simulink model "modelo_f_CAPTURAS_FINALES"  (R2024b)
settings: Solver=ode15s  StartTime=0.0  StopTime=50  FixedStep=T_s  RelTol=1e-3
InitFcn:
  | clc
  | clear
  | close all
  | clear all
  | clear mex
  | parametros
  | gain_CL
  | calculo_observador_carro
  | calculo_observador_izaje
values from neighbouring files (symbols this model uses):
  b_cx = 1e6    (= 1000000)    [parametros.m]
  b_cy = 1e7    (= 10000000)    [parametros.m]
  b_hb = 1e8    (= 100000000)    [parametros.m]
  b_hd = 8    [parametros.m]
  b_hm = 18    [parametros.m]
  b_t = 90    [parametros.m]
  b_ta = M_tEq*w_des_t*(1+n_t+n_t^2)-b_tEq    [gain_CL.m]
  b_tb = 5e6    (= 5000000)    [parametros.m]
  b_td = 1.8    [parametros.m]
  b_tm = 6    [parametros.m]
  b_tw = 3e3    (= 3000)    [parametros.m]
  b_wu = 150    [parametros.m]
  container_pillars = container_pillars(randperm(19))    [parametros.m]
  dx_grid_lidar = 0.01    [parametros.m]
  escenario = 1    [parametros.m]
  g = 9.80665    [parametros.m]
  H_c = 2.59    [parametros.m]
  H_truck = 1    [parametros.m]
  i_h = 22    [parametros.m]
  i_t = 30    [parametros.m]
  J_hd_hEb = 3800    [parametros.m]
  J_hm_hb = 30    [parametros.m]
  J_td = 1200    [parametros.m]
  J_tm_tb = 7    [parametros.m]
  K_cy = 1.8e9    (= 1800000000)    [parametros.m]
  k_tsa = M_tEq*w_des_t^2*n_t*(1+n_t+n_t^2)    [gain_CL.m]
  k_tsia = M_tEq*w_des_t^3*n_t^3    [gain_CL.m]
  K_tw = 4.8e5    (= 480000)    [parametros.m]
  k_wu = 2.36e8    (= 236000000)    [parametros.m]
  Kp_ext_carro = 0.11    [gain_CL.m]
  Kp_ext_izaje = 0.5    [gain_CL.m]
  l_h0 = (Y_t0-y_l0)    (= 15)    [parametros.m]
  l_h_max = Y_t0-y_h_min    (= 65)    [parametros.m]
  l_h_maxE = l_h_max+0.5    (= 65.5)    [parametros.m]
  l_h_min = Y_t0-y_h_max    (= 5)    [parametros.m]
  l_h_minE = l_h_min-0.5    (= 4.5)    [parametros.m]
  Lt = place(At', Ct', polos_deseados)'    [calculo_observador_carro.m]
  M_cmax = 50000    [parametros.m]
  M_cmin = 2000    [parametros.m]
  M_s = 15000    [parametros.m]
  M_t = 30000    [parametros.m]
  r_hd = 0.75    [parametros.m]
  r_td = 0.50    (= 0.5)    [parametros.m]
  T_hbMax = 5e4    (= 50000)    [parametros.m]
  T_hEbMax = 1.1e6    (= 1100000)    [parametros.m]
  T_hmMax = 2e4    (= 20000)    [parametros.m]
  T_s = 0.001    [parametros.m]
  T_s0 = 0.001    [parametros.m]
  T_s1 = 0.020    (= 0.02)    [parametros.m]
  T_s2 = 0.020    (= 0.02)    [parametros.m]
  T_tbMax = 5e3    (= 5000)    [parametros.m]
  T_tmMax = 4e3    (= 4000)    [parametros.m]
  tau_tm = 1e-3    (= 0.001)    [parametros.m]
  theta_hm0 = -l_h0*i_h*2/r_hd    (= -880)    [parametros.m]
  theta_tm0 = (x_t0)*i_t/r_td    (= -1500)    [parametros.m]
  trucks0 = [0, 0, 0, 0, 0]    [parametros.m]
  v_h_max_load = 1.5    [parametros.m]
  v_h_max_noload = 3    [parametros.m]
  v_lx0 = 0    [parametros.m]
  v_ly0 = 0    [parametros.m]
  v_t0 = 0    [parametros.m]
  v_t_max = 4    [parametros.m]
  W_c = ctrb(A, B_c(:,1))    [CyO_carro.m]    (also in CyO_izaje.m; parametros.m = 2.44)
  w_hm0 = 0    [parametros.m]
  w_hm_min_BRK = 0.005    [parametros.m]
  w_hm_rated = v_h_max_load*2*i_h/r_hd    (= 88)    [parametros.m]
  w_tm0 = (v_t0)*i_t/r_td    (= 0)    [parametros.m]
  w_tm_min_BRK = 0.005    [parametros.m]
  x_c0_left = -35    [parametros.m]
  x_c0_right = 55    [parametros.m]
  x_containers_left_lim = 1.5    [parametros.m]
  x_containers_right_lim = 48.5    [parametros.m]
  x_l0 = x_t0    (= -25)    [parametros.m]
  x_lidar_offset = 3.0    (= 3)    [parametros.m]
  x_t0 = -25    [parametros.m]
  x_t_max = 50    [parametros.m]
  x_t_maxE = x_t_max+0.5    (= 50.5)    [parametros.m]
  x_t_min = -30    [parametros.m]
  x_t_minE = x_t_min-0.5    (= -30.5)    [parametros.m]
  y_h_min = -20    [parametros.m]
  y_l0 = 30    [parametros.m]
  Y_sb = 5.0    (= 5)    [parametros.m]
  Y_t0 = 45    [parametros.m]
undefined symbols (not defined in the file or in its folder): Lh, parametros
libraries: dspnetwork x2, dspsigops x1, simulink x1
(part 2 of 5)

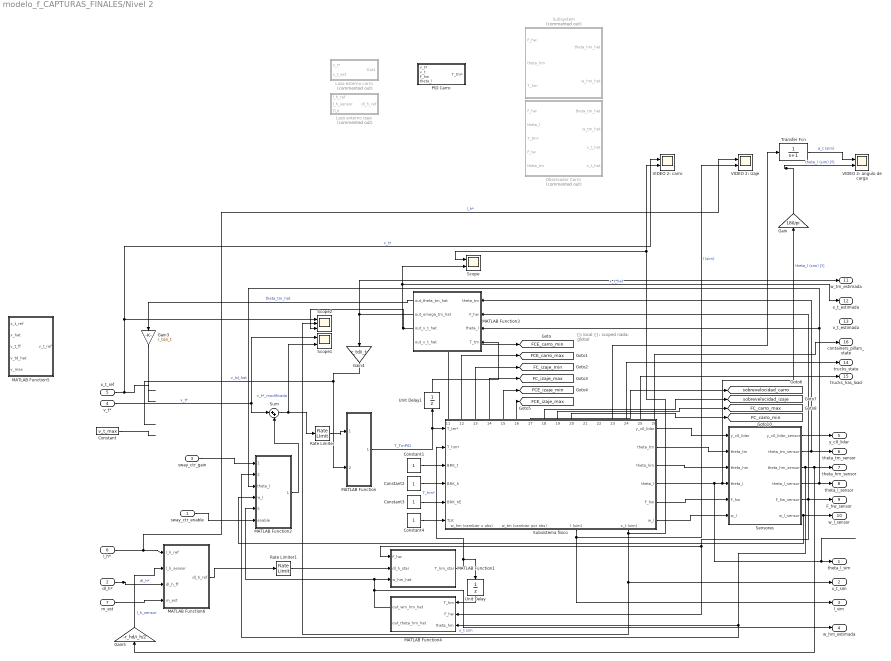
== system modelo_f_CAPTURAS_FINALES/Nivel 2 ==
  note: []: local
      | {}: scoped
      | nada: global
  sway_ctr_enable : Inport
  dl_h* : Inport  Port=2
  sway_ctr_gain : Inport  Port=3
  v_t* : Inport  Port=4
  x_t_ref : Inport  Port=5
  l_h* : Inport  Port=6
  m_est : Inport  Port=7
  Constant : Constant  Value=v_t_max
  Constant{1..4} (4 alike) : Constant
  Gain : Gain  Gain=180/pi
  Gain3 : Gain  Gain=r_td/i_t
  Gain4 : Gain  Gain=r_td/i_t
  Gain5 : Gain  Gain=-r_hd/i_h/2
  Lazo externo carro : Subsystem  Commented=on
  Lazo externo izaje : Subsystem  Commented=on
  MATLAB Function : MATLAB Function  TreatAsAtomicUnit=on  SystemSampleTime=T_s0
  MATLAB Function1 : MATLAB Function  TreatAsAtomicUnit=on  SystemSampleTime=T_s0
  MATLAB Function2 : MATLAB Function  TreatAsAtomicUnit=on  SystemSampleTime=T_s0
  MATLAB Function3 : MATLAB Function  TreatAsAtomicUnit=on  SystemSampleTime=T_s0
  MATLAB Function4 : MATLAB Function  TreatAsAtomicUnit=on  SystemSampleTime=T_s0
  MATLAB Function5 : MATLAB Function  TreatAsAtomicUnit=on
  MATLAB Function6 : MATLAB Function  TreatAsAtomicUnit=on
  Observador Carro : Subsystem  Commented=on
  PID Carro : Subsystem
  Rate Limiter : RateLimiter  RisingSlewLimit=0.8  FallingSlewLimit=-0.8  SampleTimeMode=inherited  InitialCondition=T_s
  Rate Limiter1 : RateLimiter  RisingSlewLimit=0.75  FallingSlewLimit=-0.75  SampleTimeMode=inherited  InitialCondition=T_s
  Scope : Scope  NumInputPorts=2
  Scope1 : Scope  NumInputPorts=2
  Scope2 : Scope  NumInputPorts=3
  Sensores : Subsystem
  Subsistema físico : Subsystem
      settings: PortSchema="{\"entries\":[{\"content\":{\"sides\":[{\"content\":{\"connectorIds\":[\"In1\",\"In2\",\"In3\",\"In4\",\"In5\",\"In6\"]},\"type\":\"ConnectorPlacement.EquallySpacedRectSide\",\"uuid\":\"aa1cb789-2051-45a4-8cb8-6dd2078290cc\"},{\"content\":{\"connectorIds\":[\"Out1\",\"Out2\",\"Out3\",\"Out4\",\"Out5\",\"Out6\"],\"side\":\"RIGHT\"},\"type\":\"ConnectorPlacement.EquallySpacedRectSide\",\"uuid\":\"7fe62279-dd3b-46db-ba9e-e4633dcea5c6\"},{\"content\":{\"connectorIds\":[\"Out11\",\"Out12\",\"Out13\",\"Out14\",\"Out15\",\"Out16\",\"Out17\",\"Out18\",\"Out19\",\"Out20\",\"Out21\",\"Out22\",\"Out23\",\"Out24\",\"Out25\",\"Out26\"],\"side\":\"TOP\"},\"type\":\"ConnectorPlacement.EquallySpacedRectSide\",\"uuid\":\"a5663ea7-10d8-47d7-b8ed-8fbfb239b85a\"},{\"content\":{\"connectorIds\":[\"Out7\",\"Out8\",\"Out9\",\"Out10\"],\"side\":\"BOTTOM\"},\"type\":\"ConnectorPlacement.EquallySpacedRectSide\",\"uuid\":\"9ec9131f-7b2f-42d7-8a86-9462c3c282b3\"}]},\"type\":\"ConnectorPlacement.EquallySpacedConnector\",\"uuid\":\"e7df1a56-7803-4e0d-8bf9-081877eb8c08\"}],\"packageUris\":[\"http://schema.mathworks.com/mf0/Connector/R2020b\"],\"version\":\"1.0\"}"
  Subsystem : Subsystem  Commented=on
  Sum : Sum  Inputs=|++
  Transfer Fcn : TransferFcn  Denominator=[1 1]
  Unit Delay : UnitDelay  SampleTime=T_s  HasFrameUpgradeWarning=on
  Unit Delay1 : UnitDelay  SampleTime=T_s  HasFrameUpgradeWarning=on
  VIDEO 2: angulo de carga : Scope  NumInputPorts=2
  VIDEO 2: carro : Scope  NumInputPorts=2
  VIDEO 2: izaje : Scope  NumInputPorts=2
  theta_l_sim : Outport
  x_t_sim : Outport  Port=2
  l_sim : Outport  Port=3
  w_hm_estimada : Outport  Port=4
  y_c0_lidar : Outport  Port=5
  theta_tm_sensor : Outport  Port=6
  theta_hm_sensor : Outport  Port=7
  theta_l_sensor : Outport  Port=8
  F_hw_sensor : Outport  Port=9
  w_l_sensor : Outport  Port=10
  w_tm_estimada : Outport  Port=11
  x_t_estimada : Outport  Port=12
  v_t_estimada : Outport  Port=13
  trucks_state : Outport  Port=14
  trucks_has_load : Outport  Port=15
  containers_pillars_state : Outport  Port=16
  tag scope: FCE_carro_max=global, FCE_carro_min=global, FCE_izaje_max=global, FCE_izaje_min=global, FC_carro_max=global, FC_carro_min=global, FC_izaje_max=global, FC_izaje_min=global, sobrevelocidad_carro=global, sobrevelocidad_izaje=global
  wires:
  Sensores/5(F_hw_sensor) -> F_hw_sensor/1, MATLAB Function4/2(F_hw), MATLAB Function1/1(F_hw), MATLAB Function3/2(F_hw)
  Sensores/2(theta_tm_sensor) -> theta_tm_sensor/1, MATLAB Function3/1(theta_tm)
  Subsistema físico/19(FC_carro_max) -> [FC_carro_max]
  Sensores/3(theta_hm_sensor) -> theta_hm_sensor/1, Gain5/1, MATLAB Function4/3(theta_hm), MATLAB Function2/2(theta_hm)
  Sensores/6(w_l_sensor) -> w_l_sensor/1, MATLAB Function2/4(w_l)
  Subsistema físico/15(FCE_izaje_min) -> [FCE_izaje_min]
  Unit Delay/1 -> MATLAB Function4/1(T_hm)
  Subsistema físico/13(FC_izaje_min) -> [FC_izaje_min]
  Subsistema físico/16(FCE_izaje_max) -> [FCE_izaje_max]
  MATLAB Function1/1(T_hm_star) -> Unit Delay/1, Subsistema físico/2(T_hm*)  "T_hm*"
  Subsistema físico/6(w_l) -> Sensores/6(w_l)
  Subsistema físico/17(sobrevelocidad_carro) -> [sobrevelocidad_carro]
  Subsistema físico/3(theta_hm) -> Sensores/3(theta_hm)
  MATLAB Function4/1(out_wm_hm_hat) -> MATLAB Function2/5(w_hm_hat), MATLAB Function1/3(w_hm_hat), w_hm_estimada/1
  dl_h*/1 -> MATLAB Function6/3(dl_h_ff)  "dl_h*"
  Subsistema físico/1(y_c0_lidar) -> Sensores/1(y_c0_lidar)
  Subsistema físico/5(F_hw) -> Sensores/5(F_hw)
  Subsistema físico/2(theta_tm) -> Sensores/2(theta_tm)
  Subsistema físico/18(sobrevelocidad_izaje) -> [sobrevelocidad_izaje]
  Subsistema físico/11(FCE_carro_min) -> [FCE_carro_min]
  Subsistema físico/4(theta_l) -> Gain/1, Sensores/4(theta_l), theta_l_sim/1  "theta_l (sim) [º]"
  Subsistema físico/14(FC_izaje_max) -> [FC_izaje_max]
  Subsistema físico/20(FC_carro_min) -> [FC_carro_min]
  Subsistema físico/12(FCE_carro_max) -> [FCE_carro_max]
  Constant1/1 -> Subsistema físico/3(BRK_t)
  Constant2/1 -> Subsistema físico/4(BRK_h)
  Constant3/1 -> Subsistema físico/5(BRK_hE)
  Constant4/1 -> Subsistema físico/6(TLK)
  Sensores/1(y_c0_lidar_sensor) -> y_c0_lidar/1
  sway_ctr_enable/1 -> MATLAB Function2/6(enable)
  MATLAB Function3/2(out_omega_tm_hat) -> w_tm_estimada/1, Gain4/1
  Gain4/1 -> MATLAB Function/2(v_td_hat)  "v_td_hat"
  v_t*/1 -> Sum/1, Scope1/1  "v_t*"
  Sensores/4(theta_l_sensor) -> theta_l_sensor/1, MATLAB Function2/3(theta_l), MATLAB Function3/3(theta_l)
  Unit Delay1/1 -> MATLAB Function3/4(T_tm)
  Subsistema físico/10(x_t (sim)) -> Scope2/2, x_t_sim/1, Scope/1, VIDEO 2: carro/2  "x_t sim"
  Subsistema físico/9(l (sim)) -> VIDEO 2: izaje/2, l_sim/1  "l (sim)"
  MATLAB Function3/3(out_x_t_hat) -> Scope2/3, Scope/2, x_t_estimada/1  "x_t_hat"
  MATLAB Function3/1(out_theta_tm_hat) -> Gain3/1  "theta_tm_hat"
  Subsistema físico/24(trucks_state) -> trucks_state/1
  x_t_ref/1 -> Scope2/1, VIDEO 2: carro/1  "x_t*"
  sway_ctr_gain/1 -> MATLAB Function2/1(sway_ctr_gain)
  Subsistema físico/25(trucks_has_load) -> trucks_has_load/1
  MATLAB Function/1(T_tm_star) -> Unit Delay1/1, Subsistema físico/1(T_tm*)  "T_TmPID"
  MATLAB Function2/1(v_balanceo) -> Sum/2
  Sum/1 -> Scope1/2, Rate Limiter/1  "v_t*_modificada"
  Constant/1 -> ?
  Gain3/1 -> ?
  Gain5/1 -> MATLAB Function6/2(l_h_sensor)  "l_h_sensor"
  l_h*/1 -> VIDEO 2: izaje/1, MATLAB Function6/1(l_h_ref)  "l_h*"
  MATLAB Function6/1(dl_h_ref) -> Rate Limiter1/1
  Rate Limiter/1 -> MATLAB Function/1(v_t_star)
  Rate Limiter1/1 -> MATLAB Function1/2(dl_h_star)
  Subsistema físico/26(containers_pillars_state) -> containers_pillars_state/1
  m_est/1 -> MATLAB Function6/4(m_est)
  Gain/1 -> VIDEO 2: angulo de carga/2  "theta_l (sim) [º]"
  Subsistema físico/23(a_t(sim)) -> Transfer Fcn/1
  Transfer Fcn/1 -> VIDEO 2: angulo de carga/1  "a_t (sim)"

== system modelo_f_CAPTURAS_FINALES/UDP: Controller reader ==
  Cast To Boolean{,2..5} (5 alike) : DataTypeConversion  OutDataTypeStr=boolean  SaturateOnIntegerOverflow=off  RndMeth=Floor
  MATLAB Function : MATLAB Function  TreatAsAtomicUnit=on
  UDP Receive1 : dspnetwork/UDP Receive  localURL='0.0.0.0'  localPort=5005  remoteURL='0.0.0.0'  remotePort=-1  recvBufferSize=14  dims=255  signalDatatype=uint8  isComplex=off  isVarSize=on  showBlockingTime=off  blockingTime=0  sampletime=1  blockPlatform=[]
      settings: LibrarySourceBlock=dspsrcs4/UDP Receive
  tag scope: JS_emgy_ack_cmd=global, JS_emgy_cmd=global, JS_hoist_cmd=global, JS_sway_ctrl_cmd=global, JS_system_enable=global, JS_tlk_cmd=global, JS_trolley_cmd=global
  wires:
  UDP Receive1/1 -> MATLAB Function/1(data)
  MATLAB Function/1(trolley_cmd) -> [JS_trolley_cmd]  "trolley_cmd"
  MATLAB Function/2(hoist_cmd) -> [JS_hoist_cmd]  "hoist_cmd"
  MATLAB Function/3(system_on) -> Cast To Boolean/1  "system_on"
  MATLAB Function/4(twistlock) -> Cast To Boolean2/1  "twistlock"
  MATLAB Function/5(sway_ctrl) -> Cast To Boolean3/1  "sway_ctrl"
  MATLAB Function/6(emergency) -> Cast To Boolean4/1  "emergency"
  MATLAB Function/7(emgy_ack) -> Cast To Boolean5/1  "emgy ack"
  Cast To Boolean/1 -> [JS_system_enable]
  Cast To Boolean2/1 -> [JS_tlk_cmd]
  Cast To Boolean4/1 -> [JS_emgy_cmd]
  Cast To Boolean5/1 -> [JS_emgy_ack_cmd]
  Cast To Boolean3/1 -> [JS_sway_ctrl_cmd]

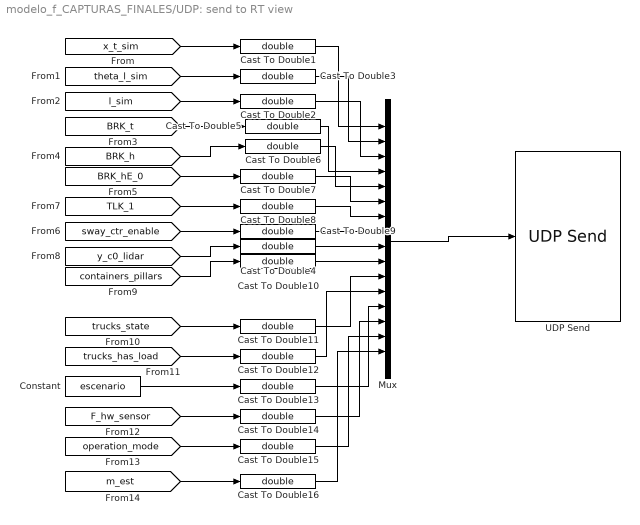
== system modelo_f_CAPTURAS_FINALES/UDP: send to RT view ==
  Cast To Double{1..16} (16 alike) : DataTypeConversion  OutDataTypeStr=double  SaturateOnIntegerOverflow=off  RndMeth=Floor
  Constant : Constant  Value=escenario
  Mux : Mux  Inputs=16
  UDP Send : dspnetwork/UDP Send  remoteURL='127.0.0.1'  remotePort=5010  localURL='0.0.0.0'  localPortSource=Automatically determine  localPort=-1  sendBufferSize=8192  sampletime=-1  blockPlatform=[]  separateLengthPort=0
      settings: LibrarySourceBlock=dspsnks4/UDP Send
  wires:
  [x_t_sim] -> Cast To Double1/1
  [theta_l_sim] -> Cast To Double3/1
  Mux/1 -> UDP Send/1
  [l_sim] -> Cast To Double2/1
  [BRK_t] -> Cast To Double5/1
  [BRK_h] -> Cast To Double6/1
  [BRK_hE_0] -> Cast To Double7/1
  [sway_ctr_enable] -> Cast To Double9/1
  [TLK_1] -> Cast To Double8/1
  Cast To Double1/1 -> Mux/1
  Cast To Double3/1 -> Mux/2
  Cast To Double2/1 -> Mux/3
  Cast To Double5/1 -> Mux/4
  Cast To Double6/1 -> Mux/5
  Cast To Double7/1 -> Mux/6
  Cast To Double8/1 -> Mux/7
  Cast To Double9/1 -> Mux/8
  [y_c0_lidar] -> Cast To Double4/1
  Cast To Double4/1 -> Mux/9
  [containers_pillars] -> Cast To Double10/1
  Cast To Double10/1 -> Mux/10
  [trucks_state] -> Cast To Double11/1
  Cast To Double11/1 -> Mux/11
  [trucks_has_load] -> Cast To Double12/1
  Cast To Double12/1 -> Mux/12
  Cast To Double13/1 -> Mux/13
  Constant/1 -> Cast To Double13/1
  Cast To Double14/1 -> Mux/14
  [F_hw_sensor] -> Cast To Double14/1
  [operation_mode] -> Cast To Double15/1
  Cast To Double15/1 -> Mux/15
  [m_est] -> Cast To Double16/1
  Cast To Double16/1 -> Mux/16

== system modelo_f_CAPTURAS_FINALES/Nivel 2/Lazo externo carro ==
  "x_t* " : Inport
  x_t_est : Inport  Port=2
  Gain : Gain  Gain=Kp_ext_carro
  Saturation : Saturate  UpperLimit=v_t_max  LowerLimit=-v_t_max
  Sum : Sum  Inputs=|+-
  Out1 : Outport
  wires:
  "x_t* "/1 -> Sum/1
  x_t_est/1 -> Sum/2
  Sum/1 -> Gain/1
  Gain/1 -> Saturation/1
  Saturation/1 -> Out1/1

== system modelo_f_CAPTURAS_FINALES/Nivel 2/Lazo externo izaje ==
  "l_h_ref " : Inport
  l_h_sensor : Inport  Port=2
  TLK : Inport  Port=3
  Gain : Gain  Gain=Kp_ext_izaje
  Sum : Sum  Inputs=|+-
  Switch : Switch  Criteria=u2 ~= 0  SaturateOnIntegerOverflow=off  InputSameDT=off
  loaded : Saturate  UpperLimit=v_h_max_load  LowerLimit=-v_h_max_load
  no load : Saturate  UpperLimit=v_h_max_noload  LowerLimit=-v_h_max_noload
  dl_h_ref : Outport
  wires:
  "l_h_ref "/1 -> Sum/1
  l_h_sensor/1 -> Sum/2
  Sum/1 -> Gain/1
  Gain/1 -> no load/1, loaded/1
  TLK/1 -> Switch/2
  loaded/1 -> Switch/1
  no load/1 -> Switch/3
  Switch/1 -> dl_h_ref/1

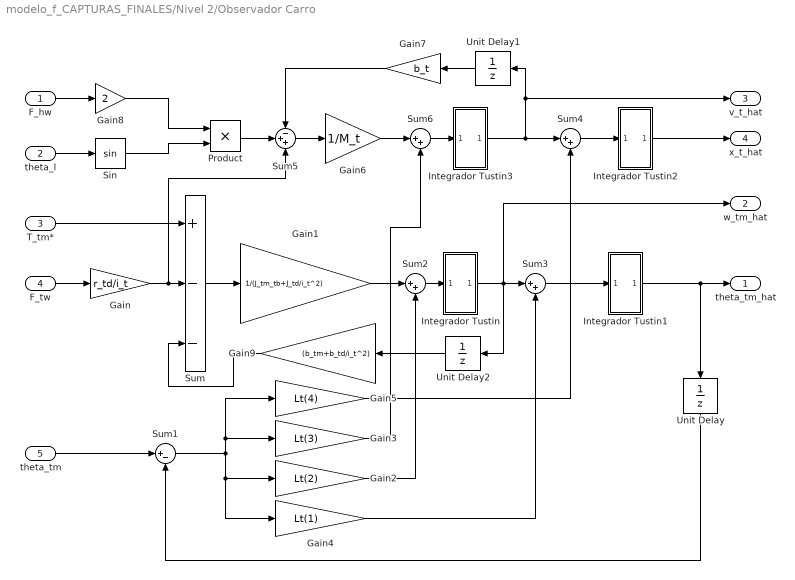
== system modelo_f_CAPTURAS_FINALES/Nivel 2/Observador Carro ==
  F_hw : Inport
  theta_l : Inport  Port=2
  T_tm* : Inport  Port=3
  F_tw : Inport  Port=4
  theta_tm : Inport  Port=5
  Gain : Gain  Gain=r_td/i_t
  Gain1 : Gain  Gain=1/(J_tm_tb+J_td/i_t^2)
  Gain2 : Gain  Gain=Lt(2)
  Gain3 : Gain  Gain=Lt(3)
  Gain4 : Gain  Gain=Lt(1)
  Gain5 : Gain  Gain=Lt(4)
  Gain6 : Gain  Gain=1/M_t
  Gain7 : Gain  Gain=b_t
  Gain8 : Gain  Gain=2
  Gain9 : Gain  Gain=(b_tm+b_td/i_t^2)
  Integrador Tustin : Subsystem
  Integrador Tustin1 : Subsystem
  Integrador Tustin2 : Subsystem
  Integrador Tustin3 : Subsystem
  Product : Product
  Sin : Trigonometry
  Sum : Sum  Inputs=+--
  Sum1 : Sum  Inputs=|+-
  Sum{2..4,6} (4 alike) : Sum  Inputs=|++
  Sum5 : Sum  Inputs=-++
  Unit Delay : UnitDelay  SampleTime=T_s1  HasFrameUpgradeWarning=on
  Unit Delay1 : UnitDelay  SampleTime=T_s1  HasFrameUpgradeWarning=on
  Unit Delay2 : UnitDelay  SampleTime=T_s1  HasFrameUpgradeWarning=on
  theta_tm_hat : Outport
  w_tm_hat : Outport  Port=2
  v_t_hat : Outport  Port=3
  x_t_hat : Outport  Port=4
  wires:
  T_tm*/1 -> Sum/1
  F_tw/1 -> Gain/1
  Gain/1 -> Sum5/3, Sum/2
  theta_tm/1 -> Sum1/1
  Integrador Tustin1/1(out) -> theta_tm_hat/1, Unit Delay/1
  Sum/1 -> Gain1/1
  Gain1/1 -> Sum2/1
  Sum2/1 -> Integrador Tustin/1(in)
  Sum3/1 -> Integrador Tustin1/1(in)
  Sum1/1 -> Gain5/1, Gain3/1, Gain2/1, Gain4/1
  Gain4/1 -> Sum3/2
  Gain2/1 -> Sum2/2
  Integrador Tustin/1(out) -> Unit Delay2/1, w_tm_hat/1, Sum3/1
  Integrador Tustin2/1(out) -> x_t_hat/1
  Sum4/1 -> Integrador Tustin2/1(in)
  Integrador Tustin3/1(out) -> Unit Delay1/1, v_t_hat/1, Sum4/1
  Gain5/1 -> Sum4/2
  Sum5/1 -> Gain6/1
  Gain7/1 -> Sum5/1
  Product/1 -> Sum5/2
  theta_l/1 -> Sin/1
  F_hw/1 -> Gain8/1
  Gain8/1 -> Product/1
  Sin/1 -> Product/2
  Gain9/1 -> Sum/3
  Unit Delay/1 -> Sum1/2
  Gain6/1 -> Sum6/1
  Sum6/1 -> Integrador Tustin3/1(in)
  Gain3/1 -> Sum6/2
  Unit Delay1/1 -> Gain7/1
  Unit Delay2/1 -> Gain9/1

== system modelo_f_CAPTURAS_FINALES/Nivel 2/PID Carro ==
  v_t* : Inport
  v_t : Inport  Port=2
  F_hw : Inport  Port=3
  theta_l : Inport  Port=4
  Gain : Gain  Gain=k_tsa
  Gain1 : Gain  Gain=k_tsia
  Gain2 : Gain  Gain=b_ta
  Gain3 : Gain  Gain=2
  Integrador Tustin1 : Subsystem
  Integrador Tustin2 : Subsystem
  Product : Product
  Sin : Trigonometry
  Sum : Sum  Inputs=|+-
  Sum1 : Sum  Inputs=+++
  Sum2 : Sum  Inputs=|+-
  T_tm* : Outport
  wires:
  v_t*/1 -> Sum/1
  v_t/1 -> Sum/2
  Sum/1 -> Gain2/1, Integrador Tustin1/1(in)
  Integrador Tustin1/1(out) -> Gain/1, Integrador Tustin2/1(in)
  Gain/1 -> Sum1/2
  Integrador Tustin2/1(out) -> Gain1/1
  Gain1/1 -> Sum1/1
  Gain2/1 -> Sum1/3
  Sum1/1 -> Sum2/1
  F_hw/1 -> Gain3/1
  theta_l/1 -> Sin/1
  Gain3/1 -> Product/1
  Sin/1 -> Product/2
  Product/1 -> Sum2/2
  Sum2/1 -> T_tm*/1

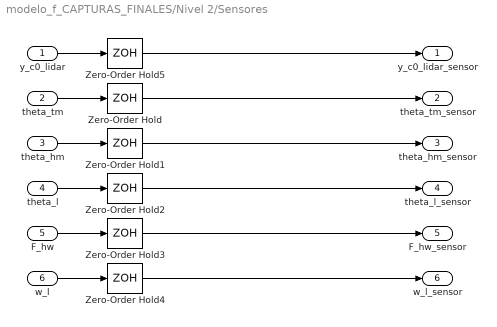
== system modelo_f_CAPTURAS_FINALES/Nivel 2/Sensores ==
  y_c0_lidar : Inport
  theta_tm : Inport  Port=2
  theta_hm : Inport  Port=3
  theta_l : Inport  Port=4
  F_hw : Inport  Port=5
  w_l : Inport  Port=6
  Zero-Order Hold{,2..5} (5 alike) : ZeroOrderHold  SampleTime=T_s
  Zero-Order Hold1 : ZeroOrderHold  SampleTime=T_s2
  y_c0_lidar_sensor : Outport
  theta_tm_sensor : Outport  Port=2
  theta_hm_sensor : Outport  Port=3
  theta_l_sensor : Outport  Port=4
  F_hw_sensor : Outport  Port=5
  w_l_sensor : Outport  Port=6
  wires:
  theta_tm/1 -> Zero-Order Hold/1
  Zero-Order Hold/1 -> theta_tm_sensor/1
  Zero-Order Hold1/1 -> theta_hm_sensor/1
  theta_hm/1 -> Zero-Order Hold1/1
  w_l/1 -> Zero-Order Hold4/1
  F_hw/1 -> Zero-Order Hold3/1
  theta_l/1 -> Zero-Order Hold2/1
  Zero-Order Hold2/1 -> theta_l_sensor/1
  Zero-Order Hold3/1 -> F_hw_sensor/1
  Zero-Order Hold4/1 -> w_l_sensor/1
  Zero-Order Hold5/1 -> y_c0_lidar_sensor/1
  y_c0_lidar/1 -> Zero-Order Hold5/1

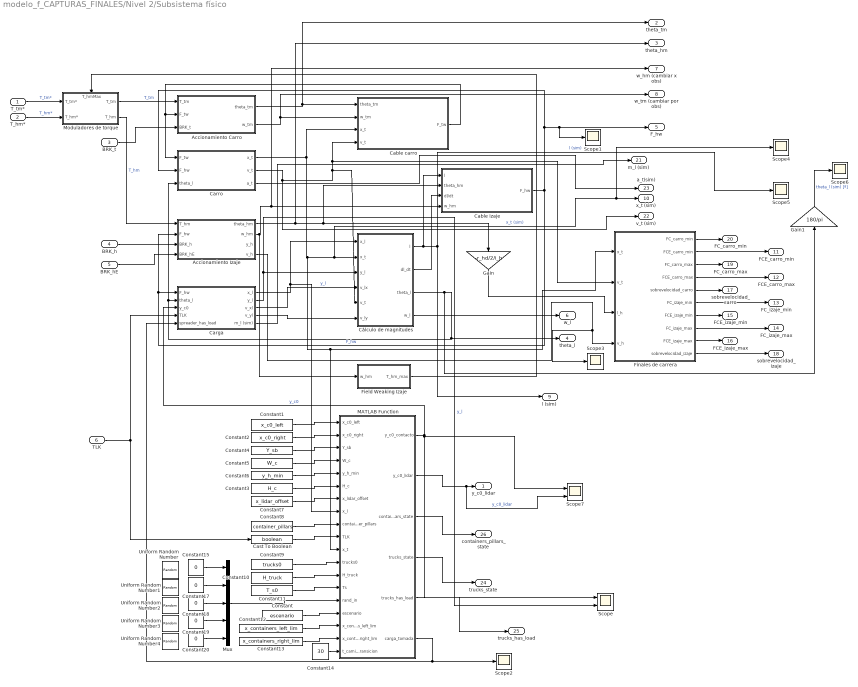
== system modelo_f_CAPTURAS_FINALES/Nivel 2/Subsistema físico ==
  T_tm* : Inport
  T_hm* : Inport  Port=2
  BRK_t : Inport  Port=3
  BRK_h : Inport  Port=4
  BRK_hE : Inport  Port=5
  TLK : Inport  Port=6
  Accionamiento Carro : Subsystem
  Accionamiento Izaje : Subsystem
  Cable carro : Subsystem
  Cable izaje : Subsystem
  Carga : Subsystem
  Carro : Subsystem
  Cast To Boolean : DataTypeConversion  OutDataTypeStr=boolean  SaturateOnIntegerOverflow=off  RndMeth=Floor
  Constant : Constant  Value=escenario
  Constant1 : Constant  Value=x_c0_left
  Constant10 : Constant  Value=H_truck
  Constant11 : Constant  Value=T_s0
  Constant12 : Constant  Value=x_containers_left_lim
  Constant13 : Constant  Value=x_containers_right_lim
  Constant14 : Constant  Value=30
  Constant{15,17..20} (5 alike) : Constant  Value=0
  Constant2 : Constant  Value=x_c0_right
  Constant3 : Constant  Value=H_c
  Constant4 : Constant  Value=Y_sb
  Constant5 : Constant  Value=W_c
  Constant6 : Constant  Value=y_h_min
  Constant7 : Constant  Value=x_lidar_offset
  Constant8 : Constant  Value=container_pillars
  Constant9 : Constant  Value=trucks0
  Cálculo de magnitudes : Subsystem
  Field Weaking Izaje : Subsystem
  Finales de carrera : Subsystem
  Gain : Gain  Gain=-r_hd/2/i_h
  Gain1 : Gain  Gain=180/pi
  MATLAB Function : MATLAB Function  TreatAsAtomicUnit=on  SystemSampleTime=T_s
  Moduladores de torque : Subsystem
      settings: PortSchema="{\"entries\":[{\"content\":{\"sides\":[{\"content\":{\"connectorIds\":[\"In1\",\"In2\"]},\"type\":\"ConnectorPlacement.EquallySpacedRectSide\",\"uuid\":\"c66d3892-523c-433a-8dde-517eb495bac1\"},{\"content\":{\"connectorIds\":[\"Out1\",\"Out2\"],\"side\":\"RIGHT\"},\"type\":\"ConnectorPlacement.EquallySpacedRectSide\",\"uuid\":\"bbb0a9b0-6ff9-4fa8-ace8-11da5b7abadd\"},{\"content\":{\"connectorIds\":[\"In3\"],\"side\":\"TOP\"},\"type\":\"ConnectorPlacement.EquallySpacedRectSide\",\"uuid\":\"35baaaad-8e6c-401a-84f7-749de5492b29\"}]},\"type\":\"ConnectorPlacement.EquallySpacedConnector\",\"uuid\":\"d8d05b6c-004b-40f1-854a-ea077232777a\"}],\"packageUris\":[\"http://schema.mathworks.com/mf0/Connector/R2020b\"],\"version\":\"1.0\"}"
  Mux : Mux  Inputs=5
  Scope : Scope  NumInputPorts=2
  Scope{1..6} (6 alike) : Scope
  Scope7 : Scope  NumInputPorts=2
  Uniform Random Number : UniformRandomNumber  Minimum=0  Seed=12415  SampleTime=T_s0
  Uniform Random Number1 : UniformRandomNumber  Minimum=0  Seed=3123  SampleTime=T_s0
  Uniform Random Number2 : UniformRandomNumber  Minimum=0  Seed=123124  SampleTime=T_s0
  Uniform Random Number3 : UniformRandomNumber  Minimum=0  Seed=28682  SampleTime=T_s0
  Uniform Random Number4 : UniformRandomNumber  Minimum=0  Seed=999  SampleTime=T_s0
  y_c0_lidar : Outport
  theta_tm : Outport  Port=2
  theta_hm : Outport  Port=3
  theta_l : Outport  Port=4
  F_hw : Outport  Port=5
  w_l : Outport  Port=6
  w_hm (cambiar x obs) : Outport  Port=7
  w_tm (cambiar por obs) : Outport  Port=8
  l (sim) : Outport  Port=9
  x_t (sim) : Outport  Port=10
  FCE_carro_min : Outport  Port=11
  FCE_carro_max : Outport  Port=12
  FC_izaje_min : Outport  Port=13
  FC_izaje_max : Outport  Port=14
  FCE_izaje_min : Outport  Port=15
  FCE_izaje_max : Outport  Port=16
  sobrevelocidad_carro : Outport  Port=17
  sobrevelocidad_izaje : Outport  Port=18
  FC_carro_max : Outport  Port=19
  FC_carro_min : Outport  Port=20
  m_l (sim) : Outport  Port=21
  v_t (sim) : Outport  Port=22
  a_t(sim) : Outport  Port=23
  trucks_state : Outport  Port=24
  trucks_has_load : Outport  Port=25
  containers_pillars_state : Outport  Port=26
  wires:
  T_tm*/1 -> Moduladores de torque/1(T_tm*)  "T_tm*"
  Accionamiento Carro/1(theta_tm) -> theta_tm/1, Cable carro/1(theta_tm)
  Accionamiento Carro/2(w_tm) -> w_tm (cambiar por obs)/1, Cable carro/2(w_tm)
  Carro/1(x_t) -> Finales de carrera/1(x_t), MATLAB Function/11(x_t), Scope4/1, x_t (sim)/1, Cálculo de magnitudes/2(x_t), Cable carro/3(x_t)  "x_t (sim)"
  Carro/2(v_t) -> v_t (sim)/1, Cálculo de magnitudes/5(v_t), Cable carro/4(v_t), Finales de carrera/2(v_t)
  Cable carro/1(F_tw) -> Carro/1(F_tw), Accionamiento Carro/2(F_tw)
  Carga/1(x_l) -> MATLAB Function/8(x_l), Cálculo de magnitudes/1(x_l)
  Carga/2(y_l) -> Scope/2, Cálculo de magnitudes/3(y_l)  "y_l"
  Carga/3(v_xl) -> Cálculo de magnitudes/4(v_lx)  "y_l"
  Carga/4(v_yl) -> Cálculo de magnitudes/6(v_ly)
  Cálculo de magnitudes/1(l) -> Scope5/1, l (sim)/1, Cable izaje/1(l)  "l (sim)"
  Accionamiento Izaje/1(theta_hm) -> Gain/1, Cable izaje/2(theta_hm), theta_hm/1
  Cálculo de magnitudes/2(dl_dt) -> Cable izaje/3(dl/dt)
  T_hm*/1 -> Moduladores de torque/2(T_hm*)  "T_hm*"
  Accionamiento Izaje/2(w_hm) -> w_hm (cambiar x obs)/1, Cable izaje/4(w_hm), Field Weaking Izaje/1(w_hm)
  BRK_t/1 -> Accionamiento Carro/3(BRK_t)
  BRK_h/1 -> Accionamiento Izaje/3(BRK_h)
  BRK_hE/1 -> Accionamiento Izaje/4(BRK_hE)
  Accionamiento Izaje/4(v_h) -> Finales de carrera/4(v_h), Scope3/1
  Cálculo de magnitudes/4(w_l) -> w_l/1
  Moduladores de torque/1(T_tm) -> Accionamiento Carro/1(T_tm)  "T_tm"
  Field Weaking Izaje/1(T_hm_max) -> Moduladores de torque/3(T_hmMax)
  Moduladores de torque/2(T_hm) -> Accionamiento Izaje/1(T_hm)  "T_hm"
  Finales de carrera/1(FC_carro_min) -> FC_carro_min/1
  Finales de carrera/2(FCE_carro_min) -> FCE_carro_min/1
  Finales de carrera/3(FC_carro_max) -> FC_carro_max/1
  Finales de carrera/4(FCE_carro_max) -> FCE_carro_max/1
  Finales de carrera/5(sobrevelocidad_carro) -> sobrevelocidad_carro/1
  Finales de carrera/7(FCE_izaje_min) -> FCE_izaje_min/1
  Finales de carrera/6(FC_izaje_min) -> FC_izaje_min/1
  Finales de carrera/8(FC_izaje_max) -> FC_izaje_max/1
  Finales de carrera/9(FCE_izaje_max) -> FCE_izaje_max/1
  Finales de carrera/10(sobrevelocidad_izaje) -> sobrevelocidad_izaje/1
  Constant1/1 -> MATLAB Function/1(x_c0_left)
  Constant2/1 -> MATLAB Function/2(x_c0_right)
  Constant3/1 -> MATLAB Function/6(H_c)
  Constant4/1 -> MATLAB Function/3(Y_sb)
  Constant5/1 -> MATLAB Function/4(W_c)
  Constant6/1 -> MATLAB Function/5(y_h_min)
  MATLAB Function/1(y_c0_contacto) -> Scope7/1, Scope/1, Carga/3(y_c0)  "y_c0"
  Constant7/1 -> MATLAB Function/7(x_lidar_offset)
  Gain/1 -> Finales de carrera/3(l_h)
  Carga/5(m_l (sim)) -> m_l (sim)/1
  Cálculo de magnitudes/3(theta_l) -> Gain1/1, Carro/3(theta_l), Carga/2(theta_l), theta_l/1
  Carro/3(a_t) -> a_t(sim)/1
  MATLAB Function/2(y_c0_lidar) -> Scope7/2, y_c0_lidar/1  "y_c0_lidar"
  Constant8/1 -> MATLAB Function/9(container_pillars)
  MATLAB Function/4(trucks_state) -> trucks_state/1
  Constant9/1 -> MATLAB Function/12(trucks0)
  Constant10/1 -> MATLAB Function/13(H_truck)
  Constant11/1 -> MATLAB Function/14(Ts)
  Constant17/1 -> Mux/2
  Constant15/1 -> Mux/1
  Constant18/1 -> Mux/3
  Constant19/1 -> Mux/4
  Constant20/1 -> Mux/5
  Constant/1 -> MATLAB Function/16(escenario)
  MATLAB Function/5(trucks_has_load) -> trucks_has_load/1
  Constant12/1 -> MATLAB Function/17(x_containers_left_lim)
  Constant13/1 -> MATLAB Function/18(x_containers_right_lim)
  MATLAB Function/3(containers_pillars_state) -> containers_pillars_state/1
  TLK/1 -> Cast To Boolean/1, Carga/4(TLK)
  Cast To Boolean/1 -> MATLAB Function/10(TLK)
  Cable izaje/1(F_hw) -> Carro/2(F_hw), Scope1/1, F_hw/1, Accionamiento Izaje/2(F_hw), Carga/1(F_hw)  "F_hw"
  MATLAB Function/6(carga_tomada) -> Scope2/1, Carga/5(spreader_has_load)
  Constant14/1 -> MATLAB Function/19(t_camion_transicion)
  Gain1/1 -> Scope6/1  "theta_l (sim) [º]"
  Mux/1 -> MATLAB Function/15(rand_in)

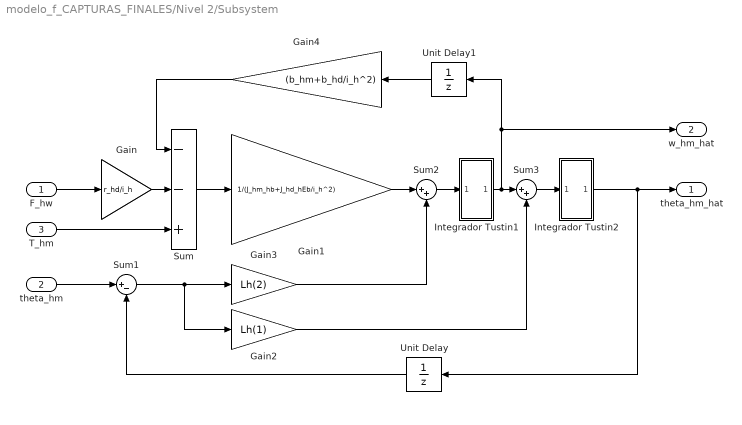
== system modelo_f_CAPTURAS_FINALES/Nivel 2/Subsystem ==
  F_hw : Inport
  theta_hm : Inport  Port=2
  T_hm : Inport  Port=3
  Gain : Gain  Gain=r_hd/i_h
  Gain1 : Gain  Gain=1/(J_hm_hb+J_hd_hEb/i_h^2)
  Gain2 : Gain  Gain=Lh(1)
  Gain3 : Gain  Gain=Lh(2)
  Gain4 : Gain  Gain=(b_hm+b_hd/i_h^2)
  Integrador Tustin1 : Subsystem
  Integrador Tustin2 : Subsystem
  Sum : Sum  Inputs=--+
  Sum1 : Sum  Inputs=|+-
  Sum2 : Sum  Inputs=|++
  Sum3 : Sum  Inputs=|++
  Unit Delay : UnitDelay  SampleTime=T_s1  HasFrameUpgradeWarning=on
  Unit Delay1 : UnitDelay  SampleTime=T_s1  HasFrameUpgradeWarning=on
  theta_hm_hat : Outport
  w_hm_hat : Outport  Port=2
  wires:
  Gain4/1 -> Sum/1
  F_hw/1 -> Gain/1
  Gain/1 -> Sum/2
  theta_hm/1 -> Sum1/1
  Sum/1 -> Gain1/1
  Gain1/1 -> Sum2/1
  Sum2/1 -> Integrador Tustin1/1(in)
  Gain3/1 -> Sum2/2
  Integrador Tustin1/1(out) -> Unit Delay1/1, w_hm_hat/1, Sum3/1
  Sum3/1 -> Integrador Tustin2/1(in)
  Gain2/1 -> Sum3/2
  Sum1/1 -> Gain2/1, Gain3/1
  Integrador Tustin2/1(out) -> theta_hm_hat/1, Unit Delay/1
  T_hm/1 -> Sum/3
  Unit Delay/1 -> Sum1/2
  Unit Delay1/1 -> Gain4/1

== system modelo_f_CAPTURAS_FINALES/Nivel 2/Observador Carro/Integrador Tustin ==
  in : Inport
  Delay : Delay  DelayLength=1  InputProcessing=Columns as channels (frame based)  SampleTime=T_s2
  Delay1 : Delay  DelayLength=1  InputProcessing=Columns as channels (frame based)  SampleTime=T_s2
  Gain : Gain  Gain=T_s2/2
  Sum : Sum  Inputs=|++
  Sum1 : Sum  Inputs=|++
  out : Outport
  wires:
  in/1 -> Sum/1, Delay/1
  Delay/1 -> Sum/2
  Sum/1 -> Gain/1
  Gain/1 -> Sum1/1
  Delay1/1 -> Sum1/2
  Sum1/1 -> out/1, Delay1/1

== system modelo_f_CAPTURAS_FINALES/Nivel 2/Observador Carro/Integrador Tustin1 ==
  in : Inport
  Delay : Delay  DelayLength=1  InputProcessing=Columns as channels (frame based)  SampleTime=T_s2
  Delay1 : Delay  DelayLength=1  InputProcessing=Columns as channels (frame based)  SampleTime=T_s2
  Gain : Gain  Gain=T_s2/2
  Sum : Sum  Inputs=|++
  Sum1 : Sum  Inputs=|++
  out : Outport
  wires:
  in/1 -> Sum/1, Delay/1
  Delay/1 -> Sum/2
  Sum/1 -> Gain/1
  Gain/1 -> Sum1/1
  Delay1/1 -> Sum1/2
  Sum1/1 -> out/1, Delay1/1

== system modelo_f_CAPTURAS_FINALES/Nivel 2/Observador Carro/Integrador Tustin2 ==
  in : Inport
  Delay : Delay  DelayLength=1  InputProcessing=Columns as channels (frame based)  SampleTime=T_s2
  Delay1 : Delay  DelayLength=1  InputProcessing=Columns as channels (frame based)  SampleTime=T_s2
  Gain : Gain  Gain=T_s2/2
  Sum : Sum  Inputs=|++
  Sum1 : Sum  Inputs=|++
  out : Outport
  wires:
  in/1 -> Sum/1, Delay/1
  Delay/1 -> Sum/2
  Sum/1 -> Gain/1
  Gain/1 -> Sum1/1
  Delay1/1 -> Sum1/2
  Sum1/1 -> out/1, Delay1/1

== system modelo_f_CAPTURAS_FINALES/Nivel 2/Observador Carro/Integrador Tustin3 ==
  in : Inport
  Delay : Delay  DelayLength=1  InputProcessing=Columns as channels (frame based)  SampleTime=T_s2
  Delay1 : Delay  DelayLength=1  InputProcessing=Columns as channels (frame based)  SampleTime=T_s2
  Gain : Gain  Gain=T_s2/2
  Sum : Sum  Inputs=|++
  Sum1 : Sum  Inputs=|++
  out : Outport
  wires:
  in/1 -> Sum/1, Delay/1
  Delay/1 -> Sum/2
  Sum/1 -> Gain/1
  Gain/1 -> Sum1/1
  Delay1/1 -> Sum1/2
  Sum1/1 -> out/1, Delay1/1

== system modelo_f_CAPTURAS_FINALES/Nivel 2/PID Carro/Integrador Tustin1 ==
  in : Inport
  Delay : Delay  DelayLength=1  InputProcessing=Columns as channels (frame based)  SampleTime=T_s2
  Delay1 : Delay  DelayLength=1  InputProcessing=Columns as channels (frame based)  SampleTime=T_s2
  Gain : Gain  Gain=T_s2/2
  Sum : Sum  Inputs=|++
  Sum1 : Sum  Inputs=|++
  out : Outport
  wires:
  in/1 -> Sum/1, Delay/1
  Delay/1 -> Sum/2
  Sum/1 -> Gain/1
  Gain/1 -> Sum1/1
  Delay1/1 -> Sum1/2
  Sum1/1 -> out/1, Delay1/1

== system modelo_f_CAPTURAS_FINALES/Nivel 2/PID Carro/Integrador Tustin2 ==
  in : Inport
  Delay : Delay  DelayLength=1  InputProcessing=Columns as channels (frame based)  SampleTime=T_s2
  Delay1 : Delay  DelayLength=1  InputProcessing=Columns as channels (frame based)  SampleTime=T_s2
  Gain : Gain  Gain=T_s2/2
  Sum : Sum  Inputs=|++
  Sum1 : Sum  Inputs=|++
  out : Outport
  wires:
  in/1 -> Sum/1, Delay/1
  Delay/1 -> Sum/2
  Sum/1 -> Gain/1
  Gain/1 -> Sum1/1
  Delay1/1 -> Sum1/2
  Sum1/1 -> out/1, Delay1/1

== system modelo_f_CAPTURAS_FINALES/Nivel 2/Subsistema físico/Accionamiento Carro ==
  T_tm : Inport
  F_tw : Inport  Port=2
  BRK_t : Inport  Port=3
  Gain : Gain  Gain=1/(J_tm_tb+J_td/i_t^2)
  Gain1 : Gain  Gain=r_td/i_t
  Gain2 : Gain  Gain=(b_tm+b_td/i_t^2)
  Integrator : Integrator  InitialCondition=w_tm0
  Integrator1 : Integrator  InitialCondition=theta_tm0
  Subsystem : Subsystem
  Sum : Sum  Inputs=+-+-
  theta_tm : Outport
  w_tm : Outport  Port=2
  wires:
  Integrator1/1 -> theta_tm/1
  Integrator/1 -> w_tm/1, Gain2/1, Subsystem/2(w_tm), Integrator1/1  "w_tm"
  Gain/1 -> Integrator/1
  Sum/1 -> Gain/1
  T_tm/1 -> Sum/1
  F_tw/1 -> Gain1/1
  Gain1/1 -> Sum/2
  Subsystem/1(T_tb) -> Sum/3
  Gain2/1 -> Sum/4
  BRK_t/1 -> Subsystem/1(BRK_t)

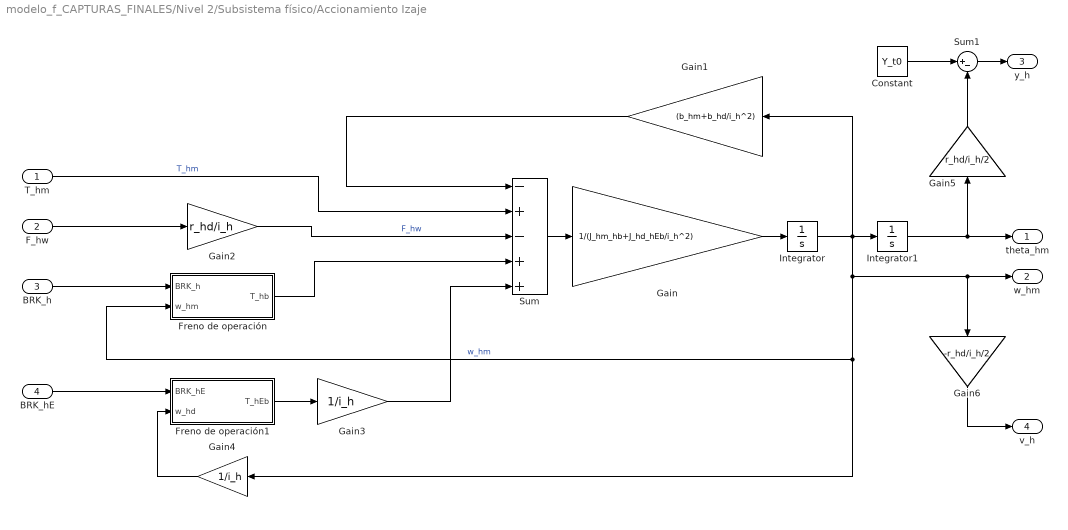
== system modelo_f_CAPTURAS_FINALES/Nivel 2/Subsistema físico/Accionamiento Izaje ==
  T_hm : Inport
  F_hw : Inport  Port=2
  BRK_h : Inport  Port=3
  BRK_hE : Inport  Port=4
  Constant : Constant  Value=Y_t0
  Freno de operación : Subsystem
  Freno de operación1 : Subsystem
  Gain : Gain  Gain=1/(J_hm_hb+J_hd_hEb/i_h^2)
  Gain1 : Gain  Gain=(b_hm+b_hd/i_h^2)
  Gain2 : Gain  Gain=r_hd/i_h
  Gain3 : Gain  Gain=1/i_h
  Gain4 : Gain  Gain=1/i_h
  Gain5 : Gain  Gain=r_hd/i_h/2
  Gain6 : Gain  Gain=-r_hd/i_h/2
  Integrator : Integrator  InitialCondition=w_hm0
  Integrator1 : Integrator  InitialCondition=theta_hm0
  Sum : Sum  Inputs=-+-++
  Sum1 : Sum  Inputs=|+-
  theta_hm : Outport
  w_hm : Outport  Port=2
  y_h : Outport  Port=3
  v_h : Outport  Port=4
  wires:
  Integrator1/1 -> Gain5/1, theta_hm/1
  Integrator/1 -> Integrator1/1, Gain6/1, w_hm/1, Gain4/1, Freno de operación/2(w_hm), Gain1/1  "w_hm"
  Gain/1 -> Integrator/1
  Sum/1 -> Gain/1
  Gain1/1 -> Sum/1
  F_hw/1 -> Gain2/1
  Gain2/1 -> Sum/3  "F_hw"
  T_hm/1 -> Sum/2  "T_hm"
  Freno de operación/1(T_hb) -> Sum/4
  BRK_h/1 -> Freno de operación/1(BRK_h)
  Freno de operación1/1(T_hEb) -> Gain3/1
  Gain3/1 -> Sum/5
  BRK_hE/1 -> Freno de operación1/1(BRK_hE)
  Gain4/1 -> Freno de operación1/2(w_hd)
  Sum1/1 -> y_h/1
  Gain5/1 -> Sum1/2
  Constant/1 -> Sum1/1
  Gain6/1 -> v_h/1

== system modelo_f_CAPTURAS_FINALES/Nivel 2/Subsistema físico/Cable carro ==
  theta_tm : Inport
  w_tm : Inport  Port=2
  x_t : Inport  Port=3
  v_t : Inport  Port=4
  Gain : Gain  Gain=b_tw
  Gain1 : Gain  Gain=K_tw
  Gain2 : Gain  Gain=r_td/i_t
  Gain3 : Gain  Gain=r_td/i_t
  Sum : Sum  Inputs=|+-
  Sum1 : Sum  Inputs=|+-
  Sum2 : Sum  Inputs=|++
  F_tw : Outport
  wires:
  Sum/1 -> Gain1/1
  theta_tm/1 -> Gain3/1
  x_t/1 -> Sum/2
  Sum1/1 -> Gain/1
  w_tm/1 -> Gain2/1
  v_t/1 -> Sum1/2
  Gain/1 -> Sum2/2
  Gain1/1 -> Sum2/1
  Sum2/1 -> F_tw/1
  Gain2/1 -> Sum1/1  "v_td"
  Gain3/1 -> Sum/1  "x_td"

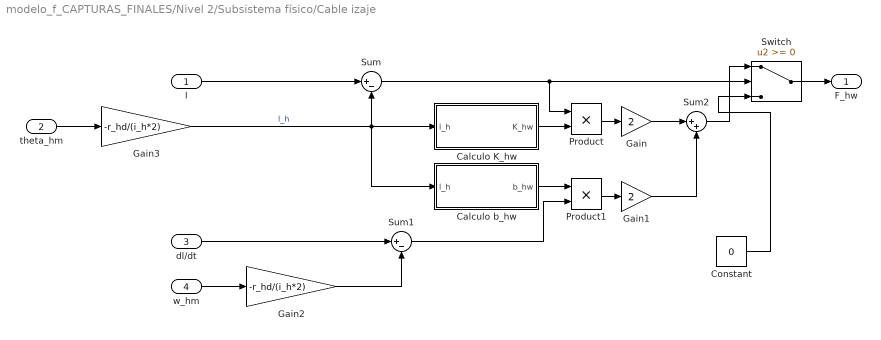
== system modelo_f_CAPTURAS_FINALES/Nivel 2/Subsistema físico/Cable izaje ==
  l : Inport
  theta_hm : Inport  Port=2
  dl/dt : Inport  Port=3
  w_hm : Inport  Port=4
  Calculo K_hw : Subsystem
  Calculo b_hw : Subsystem
  Constant : Constant  Value=0
  Gain : Gain  Gain=2
  Gain1 : Gain  Gain=2
  Gain2 : Gain  Gain=-r_hd/(i_h*2)
  Gain3 : Gain  Gain=-r_hd/(i_h*2)
  Product : Product
  Product1 : Product
  Sum : Sum  Inputs=|+-
  Sum1 : Sum  Inputs=|+-
  Sum2 : Sum  Inputs=|++
  Switch : Switch  SaturateOnIntegerOverflow=off  InputSameDT=off
  F_hw : Outport
  wires:
  l/1 -> Sum/1
  theta_hm/1 -> Gain3/1
  Sum/1 -> Product/1, Switch/2
  Calculo K_hw/1(K_hw) -> Product/2
  Product/1 -> Gain/1
  w_hm/1 -> Gain2/1
  Product1/1 -> Gain1/1
  Calculo b_hw/1(b_hw) -> Product1/1
  Gain1/1 -> Sum2/2
  Gain/1 -> Sum2/1
  Sum2/1 -> Switch/1
  Switch/1 -> F_hw/1
  dl/dt/1 -> Sum1/1
  Constant/1 -> Switch/3
  Gain2/1 -> Sum1/2
  Gain3/1 -> Calculo b_hw/1(l_h), Calculo K_hw/1(l_h), Sum/2  "l_h"
  Sum1/1 -> Product1/2

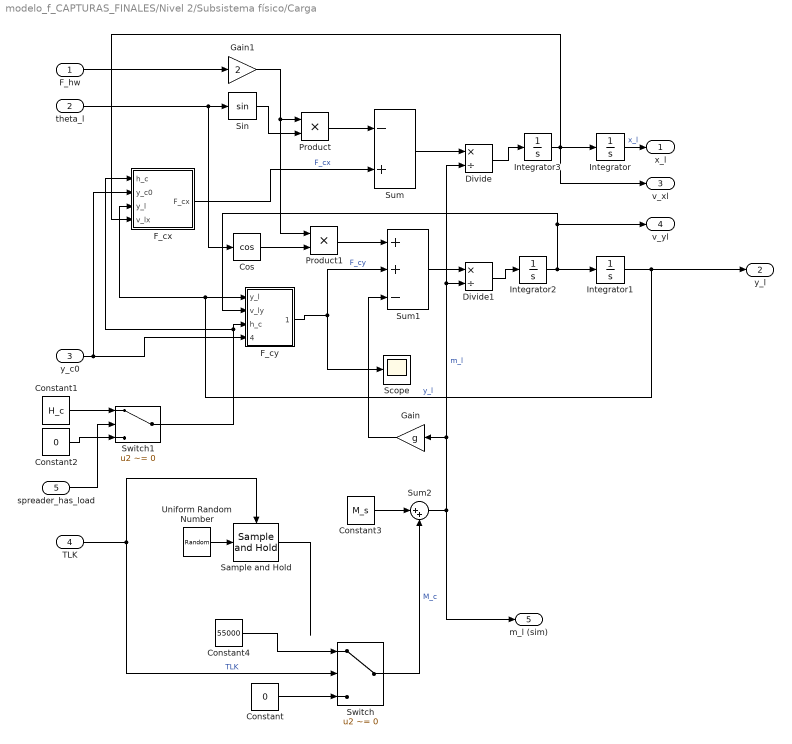
== system modelo_f_CAPTURAS_FINALES/Nivel 2/Subsistema físico/Carga ==
  F_hw : Inport
  theta_l : Inport  Port=2
  y_c0 : Inport  Port=3
  TLK : Inport  Port=4
  spreader_has_load : Inport  Port=5
  Constant : Constant  Value=0
  Constant1 : Constant  Value=H_c
  Constant2 : Constant  Value=0
  Constant3 : Constant  Value=M_s
  Constant4 : Constant  Value=55000
  Cos : Trigonometry  Operator=cos
  Divide : Product  Inputs=*/
  Divide1 : Product  Inputs=*/
  F_cx : Subsystem
  F_cy : Subsystem
  Gain : Gain  Gain=g
  Gain1 : Gain  Gain=2
  Integrator : Integrator  InitialCondition=x_l0
  Integrator1 : Integrator  InitialCondition=y_l0
  Integrator2 : Integrator  InitialCondition=v_ly0
  Integrator3 : Integrator  InitialCondition=v_lx0
  Product : Product
  Product1 : Product
  Sample and Hold : dspsigops/Sample and Hold  trig=Rising edge  initCond=0  latchinput=off
  Scope : Scope
  Sin : Trigonometry
  Sum : Sum  Inputs=-+
  Sum1 : Sum  Inputs=++-
  Sum2 : Sum  Inputs=|++
  Switch : Switch  Criteria=u2 ~= 0  SaturateOnIntegerOverflow=off  InputSameDT=off
  Switch1 : Switch  Criteria=u2 ~= 0  SaturateOnIntegerOverflow=off  InputSameDT=off
  Uniform Random Number : UniformRandomNumber  Minimum=M_cmin  Maximum=M_cmax  SampleTime=1
  x_l : Outport
  y_l : Outport  Port=2
  v_xl : Outport  Port=3
  v_yl : Outport  Port=4
  m_l (sim) : Outport  Port=5
  wires:
  Sum/1 -> Divide/1
  Divide/1 -> Integrator3/1
  theta_l/1 -> Cos/1, Sin/1
  F_hw/1 -> Gain1/1
  Gain1/1 -> Product/1, Product1/1
  Sin/1 -> Product/2
  Product/1 -> Sum/1
  Switch1/1 -> F_cx/1(h_c), F_cy/3(h_c)
  Product1/1 -> Sum1/1
  Cos/1 -> Product1/2
  F_cy/1(F_cy) -> Sum1/2, Scope/1  "F_cy"
  Divide1/1 -> Integrator2/1
  Sum1/1 -> Divide1/1
  Integrator/1 -> x_l/1  "x_l"
  Integrator3/1 -> v_xl/1, F_cx/4(v_lx), Integrator/1
  Integrator2/1 -> v_yl/1, F_cy/2(v_ly), Integrator1/1
  Integrator1/1 -> y_l/1, F_cx/3(y_l), F_cy/1(y_l)  "y_l"
  y_c0/1 -> F_cx/2(y_c0), F_cy/4(y_c0)
  F_cx/1(F_cx) -> Sum/2  "F_cx"
  TLK/1 -> Sample and Hold/Trigger, Switch/2  "TLK"
  Switch/1 -> Sum2/2  "M_c"
  Constant3/1 -> Sum2/1
  Sum2/1 -> Gain/1, Divide1/2, Divide/2, m_l (sim)/1  "m_l"
  Uniform Random Number/1 -> Sample and Hold/1
  Sample and Hold/1 -> ?
  Constant/1 -> Switch/3
  Constant1/1 -> Switch1/1
  Constant2/1 -> Switch1/3
  Gain/1 -> Sum1/3
  spreader_has_load/1 -> Switch1/2
  Constant4/1 -> Switch/1

== system modelo_f_CAPTURAS_FINALES/Nivel 2/Subsistema físico/Carro ==
  F_tw : Inport
  F_hw : Inport  Port=2
  theta_l : Inport  Port=3
  Gain : Gain  Gain=2
  Gain1 : Gain  Gain=b_t
  Gain2 : Gain  Gain=1/M_t
  Integrator : Integrator  InitialCondition=v_t0
  Integrator1 : Integrator  InitialCondition=x_t0
  Product : Product
  Sin : Trigonometry
  Sum : Sum  Inputs=-++
  x_t : Outport
  v_t : Outport  Port=2
  a_t : Outport  Port=3
  wires:
  F_tw/1 -> Sum/3
  F_hw/1 -> Gain/1
  Gain/1 -> Product/1
  theta_l/1 -> Sin/1
  Sin/1 -> Product/2
  Product/1 -> Sum/2
  Integrator/1 -> v_t/1, Integrator1/1, Gain1/1  "v_t"
  Sum/1 -> Gain2/1
  Gain2/1 -> a_t/1, Integrator/1  "dv_t/dt"
  Integrator1/1 -> x_t/1
  Gain1/1 -> Sum/1

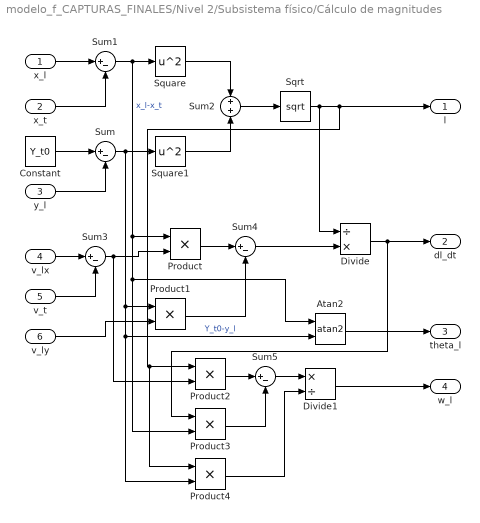
== system modelo_f_CAPTURAS_FINALES/Nivel 2/Subsistema físico/Cálculo de magnitudes ==
  x_l : Inport
  x_t : Inport  Port=2
  y_l : Inport  Port=3
  v_lx : Inport  Port=4
  v_t : Inport  Port=5
  v_ly : Inport  Port=6
  Atan2 : Trigonometry  Operator=atan2
  Constant : Constant  Value=Y_t0
  Divide : Product  Inputs=/*
  Divide1 : Product  Inputs=*/
  Product{,1..4} (5 alike) : Product
  Sqrt : Sqrt
  Square : Math  Operator=square
  Square1 : Math  Operator=square
  Sum{,1,3..5} (5 alike) : Sum  Inputs=|+-
  Sum2 : Sum  Inputs=+|+
  l : Outport
  dl_dt : Outport  Port=2
  theta_l : Outport  Port=3
  w_l : Outport  Port=4
  wires:
  Constant/1 -> Sum/1
  y_l/1 -> Sum/2
  x_l/1 -> Sum1/1
  x_t/1 -> Sum1/2
  Sum1/1 -> Product3/2, Atan2/1, Product/1, Square/1  "x_l-x_t"
  Sum/1 -> Product4/2, Atan2/2, Product1/1, Square1/1  "Y_t0-y_l"
  Square/1 -> Sum2/1
  Square1/1 -> Sum2/2
  Sum2/1 -> Sqrt/1
  Sqrt/1 -> Divide/1, Product4/1, Product2/1, l/1
  v_lx/1 -> Sum3/1
  v_t/1 -> Sum3/2
  Sum3/1 -> Product2/2, Product/2
  Product/1 -> Sum4/1
  v_ly/1 -> Product1/2
  Product1/1 -> Sum4/2
  Sum4/1 -> Divide/2
  Divide/1 -> Product3/1, dl_dt/1
  Atan2/1 -> theta_l/1
  Divide1/1 -> w_l/1
  Product2/1 -> Sum5/1
  Product3/1 -> Sum5/2
  Sum5/1 -> Divide1/1
  Product4/1 -> Divide1/2

== system modelo_f_CAPTURAS_FINALES/Nivel 2/Subsistema físico/Field Weaking Izaje ==
  w_hm : Inport
  Abs : Abs  SaturateOnIntegerOverflow=off
  Constant : Constant  Value=w_hm_rated
  Divide : Product  Inputs=*/
  Gain : Gain  Gain=T_hmMax
  Max : MinMax  Function=max  Inputs=2
  Square : Math  Operator=square
  T_hm_max : Outport
  wires:
  w_hm/1 -> Abs/1
  Constant/1 -> Divide/1, Max/2
  Divide/1 -> Square/1
  Square/1 -> Gain/1
  Gain/1 -> T_hm_max/1
  Abs/1 -> Max/1
  Max/1 -> Divide/2

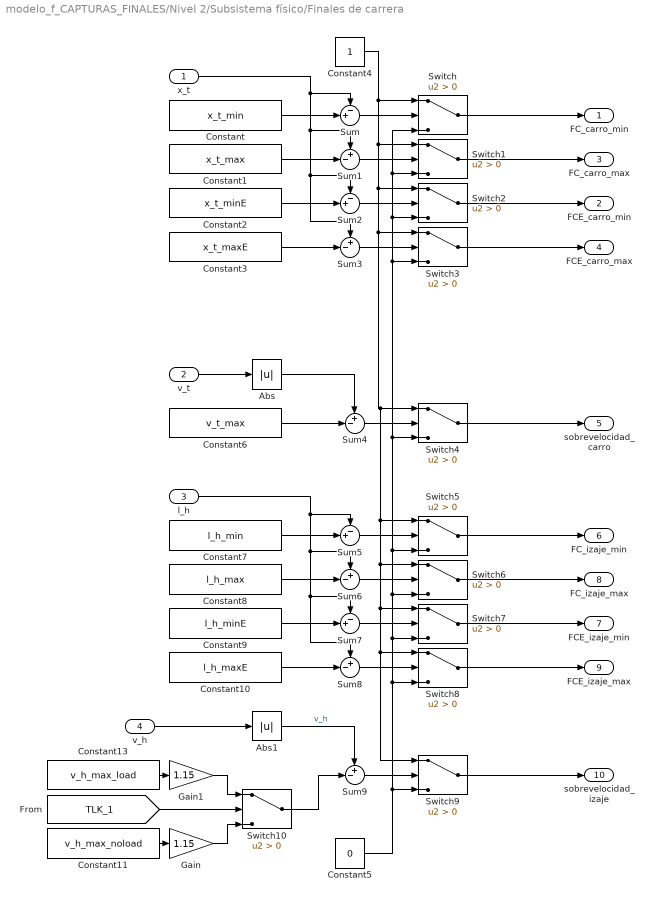
== system modelo_f_CAPTURAS_FINALES/Nivel 2/Subsistema físico/Finales de carrera ==
  x_t : Inport
  v_t : Inport  Port=2
  l_h : Inport  Port=3
  v_h : Inport  Port=4
  Abs : Abs  SaturateOnIntegerOverflow=off
  Abs1 : Abs  SaturateOnIntegerOverflow=off
  Constant : Constant  Value=x_t_min
  Constant1 : Constant  Value=x_t_max
  Constant10 : Constant  Value=l_h_maxE
  Constant11 : Constant  Value=v_h_max_noload
  Constant13 : Constant  Value=v_h_max_load
  Constant2 : Constant  Value=x_t_minE
  Constant3 : Constant  Value=x_t_maxE
  Constant4 : Constant
  Constant5 : Constant  Value=0
  Constant6 : Constant  Value=v_t_max
  Constant7 : Constant  Value=l_h_min
  Constant8 : Constant  Value=l_h_max
  Constant9 : Constant  Value=l_h_minE
  Gain : Gain  Gain=1.15
  Gain1 : Gain  Gain=1.15
  Sum{,2,5,7} (4 alike) : Sum  Inputs=-+|
  Sum{1,3..4,6,8..9} (6 alike) : Sum  Inputs=+-|
  Switch{,1..10} (11 alike) : Switch  Criteria=u2 > Threshold  SaturateOnIntegerOverflow=off  InputSameDT=off
  FC_carro_min : Outport
  FCE_carro_min : Outport  Port=2
  FC_carro_max : Outport  Port=3
  FCE_carro_max : Outport  Port=4
  sobrevelocidad_carro : Outport  Port=5
  FC_izaje_min : Outport  Port=6
  FCE_izaje_min : Outport  Port=7
  FC_izaje_max : Outport  Port=8
  FCE_izaje_max : Outport  Port=9
  sobrevelocidad_izaje : Outport  Port=10
  wires:
  Constant/1 -> Sum/2
  Constant1/1 -> Sum1/2
  Constant2/1 -> Sum2/2
  Constant3/1 -> Sum3/2
  x_t/1 -> Sum/1, Sum1/1, Sum2/1, Sum3/1
  Sum/1 -> Switch/2
  Constant4/1 -> Switch2/1, Switch9/1, Switch8/1, Switch7/1, Switch6/1, Switch5/1, Switch4/1, Switch3/1, Switch1/1, Switch/1
  Sum1/1 -> Switch1/2
  Sum2/1 -> Switch2/2
  Sum3/1 -> Switch3/2
  Switch/1 -> FC_carro_min/1
  Switch1/1 -> FC_carro_max/1
  Switch2/1 -> FCE_carro_min/1
  Switch3/1 -> FCE_carro_max/1
  v_t/1 -> Abs/1
  Constant6/1 -> Sum4/2
  Sum4/1 -> Switch4/2
  Abs/1 -> Sum4/1
  Switch4/1 -> sobrevelocidad_carro/1
  Switch7/1 -> FCE_izaje_min/1
  Switch6/1 -> FC_izaje_max/1
  l_h/1 -> Sum5/1, Sum6/1, Sum7/1, Sum8/1
  Sum7/1 -> Switch7/2
  Switch5/1 -> FC_izaje_min/1
  Constant7/1 -> Sum5/2
  Constant10/1 -> Sum8/2
  Constant9/1 -> Sum7/2
  Sum6/1 -> Switch6/2
  Constant8/1 -> Sum6/2
  Sum8/1 -> Switch8/2
  Constant5/1 -> Switch9/3, Switch8/3, Switch6/3, Switch5/3, Switch1/3, Switch/3, Switch2/3, Switch3/3, Switch4/3, Switch7/3
  Switch8/1 -> FCE_izaje_max/1
  Sum5/1 -> Switch5/2
  Constant11/1 -> Gain/1
  v_h/1 -> Abs1/1
  Abs1/1 -> Sum9/1  "v_h"
  Sum9/1 -> Switch9/2
  Switch9/1 -> sobrevelocidad_izaje/1
  Gain/1 -> Switch10/3
  [TLK_1] -> Switch10/2
  Switch10/1 -> Sum9/2
  Constant13/1 -> Gain1/1
  Gain1/1 -> Switch10/1

== system modelo_f_CAPTURAS_FINALES/Nivel 2/Subsistema físico/Moduladores de torque ==
  T_tm* : Inport
  T_hm* : Inport  Port=2
  T_hmMax : Inport  Port=3
  +-T_tmMax : Saturate  UpperLimit=+T_tmMax  LowerLimit=-T_tmMax
  Gain : Gain  Gain=1/tau_tm
  Gain1 : Gain  Gain=1/tau_tm
  Gain2 : Gain  Gain=-1
  Integrator : Integrator
  Integrator1 : Integrator
  Saturation Dynamic : simulink/Discontinuities/Saturation Dynamic  OutMin=[]  OutMax=[]  OutDataTypeStr=Inherit: Same as second input  OutDataType=fixdt(1, 16)  OutScaling=2^-10  DoSatur=off
  Sum : Sum  Inputs=|+-
  Sum1 : Sum  Inputs=|+-
  T_tm : Outport
  T_hm : Outport  Port=2
  wires:
  +-T_tmMax/1 -> T_tm/1
  Gain/1 -> Integrator/1
  Integrator/1 -> Sum/2, +-T_tmMax/1
  T_tm*/1 -> Sum/1
  Sum/1 -> Gain/1
  Gain1/1 -> Integrator1/1
  Sum1/1 -> Gain1/1
  Integrator1/1 -> Sum1/2, Saturation Dynamic/2
  T_hm*/1 -> Sum1/1
  Saturation Dynamic/1 -> T_hm/1
  T_hmMax/1 -> Gain2/1, Saturation Dynamic/1
  Gain2/1 -> Saturation Dynamic/3

== system modelo_f_CAPTURAS_FINALES/Nivel 2/Subsystem/Integrador Tustin1 ==
  in : Inport
  Delay : Delay  DelayLength=1  InputProcessing=Columns as channels (frame based)  SampleTime=T_s2
  Delay1 : Delay  DelayLength=1  InputProcessing=Columns as channels (frame based)  SampleTime=T_s2
  Gain : Gain  Gain=T_s2/2
  Sum : Sum  Inputs=|++
  Sum1 : Sum  Inputs=|++
  out : Outport
  wires:
  in/1 -> Sum/1, Delay/1
  Delay/1 -> Sum/2
  Sum/1 -> Gain/1
  Gain/1 -> Sum1/1
  Delay1/1 -> Sum1/2
  Sum1/1 -> out/1, Delay1/1

== system modelo_f_CAPTURAS_FINALES/Nivel 2/Subsystem/Integrador Tustin2 ==
  in : Inport
  Delay : Delay  DelayLength=1  InputProcessing=Columns as channels (frame based)  SampleTime=T_s2
  Delay1 : Delay  DelayLength=1  InputProcessing=Columns as channels (frame based)  SampleTime=T_s2
  Gain : Gain  Gain=T_s2/2
  Sum : Sum  Inputs=|++
  Sum1 : Sum  Inputs=|++
  out : Outport
  wires:
  in/1 -> Sum/1, Delay/1
  Delay/1 -> Sum/2
  Sum/1 -> Gain/1
  Gain/1 -> Sum1/1
  Delay1/1 -> Sum1/2
  Sum1/1 -> out/1, Delay1/1

== system modelo_f_CAPTURAS_FINALES/Nivel 2/Subsistema físico/Accionamiento Carro/Subsystem ==
  BRK_t : Inport
  w_tm : Inport  Port=2
  Constant : Constant  Value=0
  Gain : Gain  Gain=b_tb
  Gain1 : Gain  Gain=-T_tbMax
  Switch : Switch  Criteria=u2 ~= 0  SaturateOnIntegerOverflow=off  InputSameDT=off
  Tanh : Trigonometry  Operator=tanh
  T_tb : Outport
  wires:
  BRK_t/1 -> Switch/2
  Constant/1 -> Switch/1
  Gain/1 -> Tanh/1
  w_tm/1 -> Gain/1
  Switch/1 -> T_tb/1
  Tanh/1 -> Gain1/1
  Gain1/1 -> Switch/3

== system modelo_f_CAPTURAS_FINALES/Nivel 2/Subsistema físico/Accionamiento Izaje/Freno de operación ==
  BRK_h : Inport
  w_hm : Inport  Port=2
  Constant : Constant  Value=0
  Gain : Gain  Gain=b_hb
  Gain1 : Gain  Gain=-T_hbMax
  Switch : Switch  Criteria=u2 ~= 0  SaturateOnIntegerOverflow=off  InputSameDT=off
  Tanh : Trigonometry  Operator=tanh
  T_hb : Outport
  wires:
  BRK_h/1 -> Switch/2
  Constant/1 -> Switch/1
  Gain/1 -> Tanh/1
  w_hm/1 -> Gain/1
  Switch/1 -> T_hb/1
  Tanh/1 -> Gain1/1
  Gain1/1 -> Switch/3

== system modelo_f_CAPTURAS_FINALES/Nivel 2/Subsistema físico/Accionamiento Izaje/Freno de operación1 ==
  BRK_hE : Inport
  w_hd : Inport  Port=2
  Constant : Constant  Value=0
  Gain : Gain  Gain=b_hd
  Gain1 : Gain  Gain=-T_hEbMax
  Switch : Switch  Criteria=u2 ~= 0  SaturateOnIntegerOverflow=off  InputSameDT=off
  Tanh : Trigonometry  Operator=tanh
  T_hEb : Outport
  wires:
  BRK_hE/1 -> Switch/2
  Constant/1 -> Switch/1
  Gain/1 -> Tanh/1
  w_hd/1 -> Gain/1
  Switch/1 -> T_hEb/1
  Tanh/1 -> Gain1/1
  Gain1/1 -> Switch/3

== system modelo_f_CAPTURAS_FINALES/Nivel 2/Subsistema físico/Cable izaje/Calculo K_hw ==
  l_h : Inport
  Constant : Constant  Value=110
  Constant1 : Constant  Value=k_wu
  Divide : Product  Inputs=*/
  Gain : Gain  Gain=2
  Sum : Sum  Inputs=|++
  K_hw : Outport
  wires:
  l_h/1 -> Gain/1
  Gain/1 -> Sum/1
  Constant/1 -> Sum/2
  Sum/1 -> Divide/2
  Constant1/1 -> Divide/1
  Divide/1 -> K_hw/1

== system modelo_f_CAPTURAS_FINALES/Nivel 2/Subsistema físico/Cable izaje/Calculo b_hw ==
  l_h : Inport
  Constant : Constant  Value=110
  Gain : Gain  Gain=2
  Gain1 : Gain  Gain=b_wu
  Sum : Sum  Inputs=|++
  b_hw : Outport
  wires:
  l_h/1 -> Gain/1
  Gain/1 -> Sum/1
  Constant/1 -> Sum/2
  Sum/1 -> Gain1/1
  Gain1/1 -> b_hw/1

== system modelo_f_CAPTURAS_FINALES/Nivel 2/Subsistema físico/Carga/F_cx ==
  h_c : Inport
  y_c0 : Inport  Port=2
  y_l : Inport  Port=3
  v_lx : Inport  Port=4
  Constant : Constant  Value=0
  Gain : Gain  Gain=-b_cx
  Sum : Sum  Inputs=|+-
  Sum1 : Sum  Inputs=|-+
  Switch : Switch  Criteria=u2 > Threshold  SaturateOnIntegerOverflow=off  InputSameDT=off
  F_cx : Outport
  wires:
  y_l/1 -> Sum/1
  h_c/1 -> Sum/2
  Sum/1 -> Sum1/1
  y_c0/1 -> Sum1/2
  Sum1/1 -> Switch/2
  Constant/1 -> Switch/3
  v_lx/1 -> Gain/1
  Gain/1 -> Switch/1
  Switch/1 -> F_cx/1

== system modelo_f_CAPTURAS_FINALES/Nivel 2/Subsistema físico/Carga/F_cy ==
  y_l : Inport
  v_ly : Inport  Port=2
  h_c : Inport  Port=3
  y_c0 : Inport  Port=4
  Constant1 : Constant  Value=0
  Gain : Gain  Gain=K_cy
  Gain1 : Gain  Gain=b_cy
  Sum : Sum  Inputs=|+-
  Sum1 : Sum  Inputs=|-+
  Sum2 : Sum  Inputs=|+-
  Sum3 : Sum  Inputs=|-+
  switch : Switch  Criteria=u2 > Threshold  SaturateOnIntegerOverflow=off  InputSameDT=off
  F_cy : Outport
  wires:
  switch/1 -> F_cy/1
  Sum2/1 -> switch/1
  Constant1/1 -> switch/3
  Sum/1 -> Sum3/1, Sum1/1
  y_l/1 -> Sum/1
  h_c/1 -> Sum/2
  y_c0/1 -> Sum3/2, Sum1/2
  Sum1/1 -> Gain/1
  Gain/1 -> Sum2/1
  v_ly/1 -> Gain1/1
  Gain1/1 -> Sum2/2
  Sum3/1 -> switch/2

== matlab function modelo_f_CAPTURAS_FINALES/Nivel 2/MATLAB Function ==
  data: v_t_star input; T_tm_star output; v_td_hat input
function T_tm_star = PID_carro(v_t_star, v_td_hat)

    persistent int1 int2 k_tsia k_tsa b_ta T_s e_prev int1_prev e_x_t_prev;

    if isempty(int1)
        int1 = 0;
        int2 = 0;
        k_tsia = 817.1486;
        k_tsa = 4.09*10^3;
        b_ta = 4.3394*10^3;
        T_s = 0.001;
        e_prev = 0;
        int1_prev = 0;
        e_x_t_prev = 0;
    end

    e_t = v_t_star - v_td_hat;

    int1 = int1 + T_s * (e_t+e_prev)/2;
    e_prev = e_t;
    int2 = int2 + T_s * (int1+int1_prev)/2;
    int1_prev = int1;



    T_tm_star = e_t * b_ta + (int1) * k_tsa + int2 * k_tsia;

end

== matlab function modelo_f_CAPTURAS_FINALES/Nivel 2/MATLAB Function1 ==
  data: F_hw input; T_hm_star output; dl_h_star input; w_hm_hat input
function T_hm_star = fcn(F_hw, dl_h_star, w_hm_hat)

persistent int1 int2 k_hsia k_hsa b_ha T_s r_hd i_h e_prev int1_prev

if isempty(int1)

    int1 = 0;
    int2 = 0;
    k_hsia = -6.4992*10^5;
    k_hsa = -4.3987*10^5;
    b_ha = -6.7646*10^4;
    T_s = 0.001;
    r_hd = 0.75;
    i_h = 22;
    e_prev = 0;
    int1_prev = 0;

end

dl_h = w_hm_hat * (-r_hd)/(i_h*2);

e_h = dl_h_star - dl_h;

int1 = int1 + T_s * (e_h+e_prev)/2;

e_prev = e_h;

int2 = int2 + T_s * (int1+int1_prev)/2;

int1_prev = int1;

T_hm_star = F_hw*r_hd/(i_h*2) + b_ha * e_h + k_hsa * int1 + k_hsia * int2;

end
